simulink model "arm_nonlinear_sim_pi_d_cont_R2015a"  (R2015a)
settings: Solver=ode4  SolverMode=SingleTasking  StartTime=0.0  StopTime=3  FixedStep=0.001  RelTol=1e-3
values from neighbouring files (symbols this model uses):
  c = 0    [i_pd_design.m]    (also in i_pd_design_R2013a.m; i_pd_design_R2015a.m; i_pd_design_R2018a.m; i_pd_design_custom.m)
  dc = 0.5    [arm_linear_pi_d_design.m]    (also in arm_linear_pi_d_design_R2013a.m; arm_linear_pi_d_design_R2015a.m; arm_linear_pi_d_design_R2018a.m; arm_linear_pi_d_design_custom.m)
  kD = (d2*gamma_m1^2 - d1*gamma_m1*gamma_m2                    + d0*(gamma_m2^2 - gamma_m1*gamma_m3))/(gamma_m1*gamma_m2)    [arm_linear_pi_d_design.m]    (also in arm_linear_pi_d_design_R2013a.m; arm_linear_pi_d_design_R2015a.m; arm_linear_pi_d_design_R2018a.m; arm_linear_pi_d_design_custom.m)
  kI = d0/gamma_m1    [arm_linear_pi_d_design.m]    (also in arm_linear_pi_d_design_R2013a.m; arm_linear_pi_d_design_R2015a.m; arm_linear_pi_d_design_R2018a.m; arm_linear_pi_d_design_custom.m)
  kP = (d2*gamma_m1 - d0*gamma_m3)/(gamma_m1*gamma_m2)    [arm_linear_pi_d_design.m]    (also in arm_linear_pi_d_design_R2013a.m; arm_linear_pi_d_design_R2015a.m; arm_linear_pi_d_design_R2018a.m; arm_linear_pi_d_design_custom.m)
  rc = rc_deg*(pi/180)    (= 0.523598775598)    [arm_linear_pi_d_design.m]    (also in arm_linear_pi_d_design_R2013a.m; arm_linear_pi_d_design_R2015a.m; arm_linear_pi_d_design_R2018a.m; arm_linear_pi_d_design_custom.m)
undefined symbols (not defined in the file or in its folder): g, J, l, M
settings Model: CovMetricSettings=dwe  CovHtmlReporting=off  covSaveCumulativeToWorkspaceVar=off  CovSaveSingleToWorkspaceVar=off  CovExternalEMLEnable=on  Creator=kawata  LastModifiedBy=kawata
settings DataIOCC: LimitDataPoints=off  SaveFormat=Dataset
settings DebuggingCC: SFUnexpectedBacktrackingDiag=error  SFNoUnconditionalDefaultTransitionDiag=error
settings HardwareCC: ProdBitPerPointer=64  ProdLargestAtomicFloat=Float  ProdIntDivRoundTo=Zero  ProdEndianess=LittleEndian  ProdHWDeviceType=Specified
settings ModelReferenceCC: PropagateSignalLabelsOutOfModel=on
settings GRTTargetCC: TargetLangStandard=C99 (ISO)  GeneratePreprocessorConditionals=Use local settings

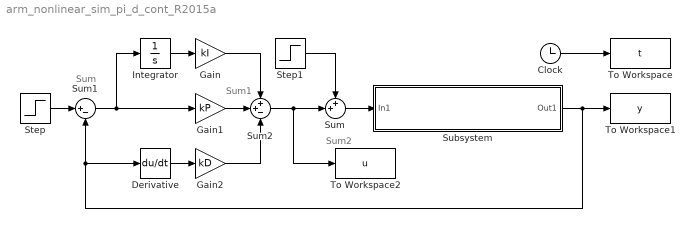
== system arm_nonlinear_sim_pi_d_cont_R2015a ==
  note: Sum1
  note: Sum2
  note: Sum
  Clock : Clock
  Derivative : Derivative
  Gain : Gain  Gain=kI
  Gain1 : Gain  Gain=kP
  Gain2 : Gain  Gain=kD
  Integrator : Integrator
  Step : Step  Time=0  After=rc  SampleTime=0
  Step1 : Step  Time=1.5  After=dc  SampleTime=0
  Subsystem : Subsystem
  Sum : Sum  Inputs=++|
  Sum1 : Sum  Inputs=|+-
  Sum2 : Sum  Inputs=++-
  To Workspace : ToWorkspace  VariableName=t  SampleTime=-1
  To Workspace1 : ToWorkspace  VariableName=y  SampleTime=-1
  To Workspace2 : ToWorkspace  VariableName=u  SampleTime=-1
  wires:
  Subsystem/1(Out1) -> To Workspace1/1, Derivative/1, Sum1/2
  Clock/1 -> To Workspace/1
  Step/1 -> Sum1/1
  Sum/1 -> Subsystem/1(In1)
  Step1/1 -> Sum/1
  Sum2/1 -> To Workspace2/1, Sum/2
  Gain1/1 -> Sum2/2
  Derivative/1 -> Gain2/1
  Gain2/1 -> Sum2/3
  Gain/1 -> Sum2/1
  Sum1/1 -> Gain1/1, Integrator/1
  Integrator/1 -> Gain/1

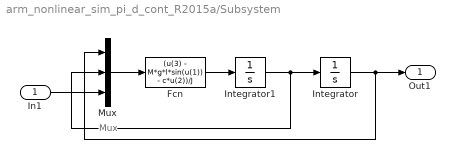
== system arm_nonlinear_sim_pi_d_cont_R2015a/Subsystem ==
  note: Mux
  In1 : Inport
  Fcn : Fcn  Expr=(u(3) - M*g*l*sin(u(1)) - c*u(2))/J
  Integrator : Integrator
  Integrator1 : Integrator
  Mux : Mux  Inputs=3
  Out1 : Outport
  wires:
  Mux/1 -> Fcn/1
  Fcn/1 -> Integrator1/1
  Integrator1/1 -> Mux/2, Integrator/1
  Integrator/1 -> Out1/1, Mux/1
  In1/1 -> Mux/3
